simulink model "test_np_gen"  (Simulink 7.7)
settings: Solver=FixedStepDiscrete  StartTime=0.0  StopTime=10000.0  FixedStep=1  RelTol=1e-3
libraries: SimpleModeling x2
settings Model: Creator=iris  LastModifiedBy=iris
settings DataIOCC: SaveFormat=StructureWithTime  SignalLogging=off
settings OptimizationCC: BlockReduction=off  ConditionallyExecuteInputs=off  InlineParams=on
settings DebuggingCC: AlgebraicLoopMsg=error
settings HardwareCC: ProdHWDeviceType=ASIC/FPGA->ASIC/FPGA

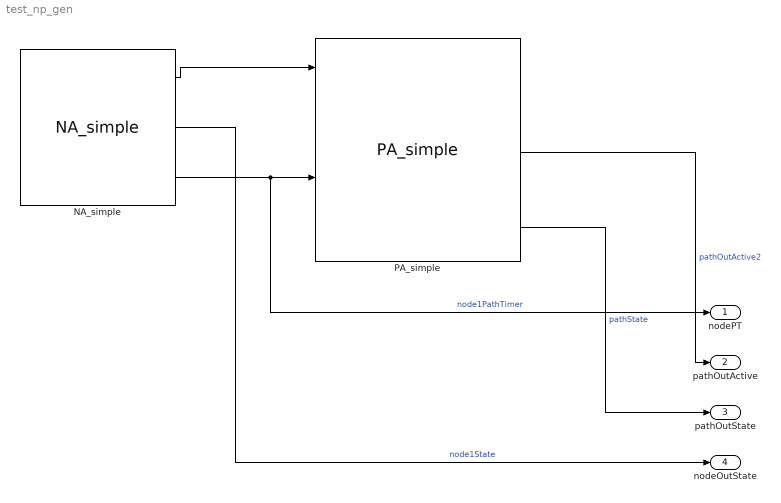
== system test_np_gen ==
  NA_simple : SimpleModeling/NA_simple  SystemSampleTime=-1  TERP_defs=0  TRRP_def=100  Trest_def=800  TERP_s=320  TRRP_s=100  Trest_s=800  Terp_min=150  Terp_max=300
  PA_simple : SimpleModeling/PA_simple  SystemSampleTime=-1  min_path_par=10  bck_param=36  forw_param=36
  nodePT : Outport
  pathOutActive : Outport  Port=2
  pathOutState : Outport  Port=3
  nodeOutState : Outport  Port=4
  wires:
  NA_simple/1 -> PA_simple/1
  NA_simple/3 -> PA_simple/3, nodePT/1  "node1PathTimer"
  PA_simple/2 -> pathOutActive/1  "pathOutActive2"
  PA_simple/3 -> pathOutState/1  "pathState"
  NA_simple/2 -> nodeOutState/1  "node1State"
